simulink library "ddm"  (R2021b)
settings: Solver=VariableStepAuto  StartTime=0.0  StopTime=10.0  RelTol=1e-3
undefined symbols (not defined in the file or in its folder): ENUM_ADASACCSTA_ERROR, ENUM_ADASACCSTA_OFF, ENUM_ADASACCSTA_STANDBY, ENUM_ADASISASTA_OFF, ENUM_ALLOWMOV_ALLOWREADY, ENUM_APS, ENUM_BRKSTA_ERROR, ENUM_BRKSTA_OFF, ENUM_BRKSTA_ON, ENUM_CHGPREACTERRSTA_OBCPRE, ENUM_DCDCFAULTSTA_ANYFAULTLV1, ENUM_DCDCFAULTSTA_ANYFAULTLV2, ENUM_DRIVETRAIN_AWD, ENUM_DRIVETRAIN_FWD, ENUM_DRIVETRAIN_RWD, ENUM_DRSEATSTA_INVALID, ENUM_EDUDRTSTA_NORMAL, ENUM_EPBSTA_APPLIED, ENUM_EPBSTA_RELEASED, ENUM_HVBATTREADYPRE_READY, ENUM_MCUWARN_LV0, ENUM_MCUWARN_LV1, ENUM_MCUWARN_LV2, ENUM_MCUWARN_LV3, ENUM_MCUWARN_NOERROR, ENUM_OBCFAULTSTA_ANYFAULT, ENUM_PAS_R2F2, ENUM_PDFAULT_BATTPDFAIL, ENUM_PDFAULT_DCDCDISABLE, ENUM_PDFAULT_MCUDISABLE, ENUM_PDFAULT_MCUDISCHRG, ENUM_POWERSTA_OFF, ENUM_POWERSTA_ON, ENUM_POWERSTA_READY, ENUM_POWERSTA_STANDBY, ENUM_PRESSINDI_LOW, ENUM_PUFAULT_BATTUPFAIL, ENUM_PUFAULT_DCDCENABLEFAIL, ENUM_PUFAULT_PRECHRGCHKFAIL, ENUM_PUFAULT_SAFETYCHKFAIL, ENUM_PUSTATE_COMPLETED, ENUM_PWRSTASW_OFF, ENUM_PWRSTASW_OFFA, ENUM_PWRSTASW_OFFCHVCHRG, ENUM_PWRSTASW_OFFCLVCHRG, ENUM_PWRSTASW_ON, ENUM_PWRSTASW_ONHVCHRG, ENUM_PWRSTASW_READY, ENUM_PWRSTASW_STANDBY, ENUM_RANGESTA_12IN, ENUM_RANGESTA_12OUT, ENUM_SHIFTCOMMAND_D, ENUM_SHIFTCOMMAND_N, ENUM_SHIFTCOMMAND_P, ENUM_SHIFTCOMMAND_R, ENUM_ZONEMALFUNLV_1ST, ENUM_ZONEMALFUNLV_2ND, ENUM_ZONEMALFUNLV_3RD, ENUM_ZONEMALFUNLV_4TH, ENUM_ZONESPDCTRLMODE_ACC ... (+832)
libraries: hcu_lib x738, $bdroot x26, simulink x7
(part 8 of 25)

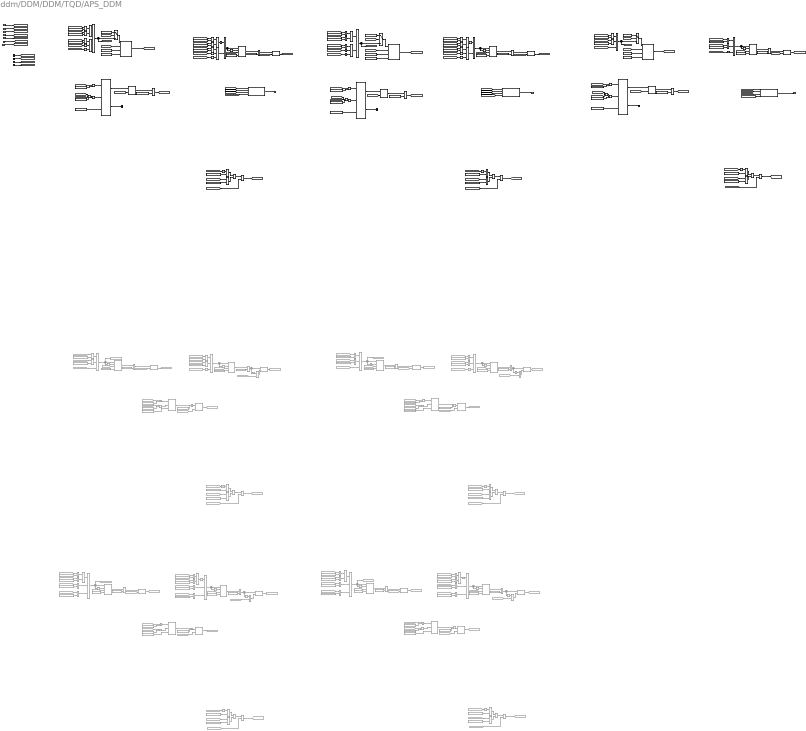
== system ddm/DDM/DDM/TQD/APS_DDM ==
  note: APS1 Signal Out of Range (APS1SigOoR)
  note: APS1_5V PWR Error (5vAPS1PwrErr)
  note: APS1 5V Out of Range (5vAPS1OoR)
  note: APS Correlation Error (APSCorrErr)
  note: APS2_5V PWR Error (5vAPS2PwrErr)
  note: APS2 Signal Out of Range (APS2SigOoR)
  note: APS2 5V Out of Range (5vAPS2OoR)
  VPMM_SysPwrSta_enum : Inport
  VINP_AccelPedal1Vol_V : Inport  Port=2
  VINP_AccelPedal2Vol_V : Inport  Port=3
  VDHP_EAPS12RangeSta_enum : Inport  Port=4
  VDHP_EAPCRBAD_flg : Inport  Port=5
  task_time_s : Inport  Port=6
  DTC_clear_request : Inport  Port=7
  Constant1 : Constant  Commented=on  Value=KDDM_5vAPS1PwrErrPassTO_ms
  Constant10 : Constant  Value=ENUM_POWERSTA_OFF
  Constant{62,65,84,92,100,103} (6 alike) : Constant  Value=ENUM_PWRSTASW_OFF
  Constant101 : Constant  Value=KDDM_APS2SigOoRHiLim_V
  Constant102 : Constant  Value=KDDM_APS2SigOoRLoLim_V
  Constant104 : Constant  Value=KDDM_APS2SigOoRHiLim_V
  Constant105 : Constant  Value=KDDM_APS2SigOoRLoLim_V
  Constant107 : Constant  Value=KDDM_APS2SigOoRPassTO_s
  Constant108 : Constant  Value=KDDM_APS2SigOoRPassTO_s
  Constant11 : Constant  Value=ENUM_POWERSTA_STANDBY
  Constant110 : Constant  Value=KDDM_APS2SigOoRCFSSW_flg
  Constant{16,20,22,72,75,79,82,111} (8 alike) : Constant  Commented=on  Value=KDDM_5vAPSErrBattSOC_pct
  Constant{9,21,32,42,44,54,112,114} (8 alike) : Constant  Commented=on  Value=ENUM_PWRSTASW_OFF
  Constant113 : Constant  Commented=on  Value=KDDM_5vAPS2PwrErrPassTO_ms
  Constant12 : Constant  Value=KDDM_APS1SigOoRDetSW_flg
  Constant13 : Constant  Value=KDDM_APS1SigOoRPassSW_flg
  Constant132 : Constant  Value=KDDM_APS1SigOoRDTC_cnt
  Constant14 : Constant  Value=KDDM_APS1SigOoRDTC_cnt
  Constant15 : Constant  Value=KDDM_APS2SigOoRDTC_cnt
  Constant17 : Constant  Commented=on  Value=KDDM_5vAPS1PwrErrDetTO_ms
  Constant18 : Constant  Commented=on  Value=KDDM_5vAPS1PwrErrDetTO_ms
  Constant19 : Constant  Commented=on  Value=KDDM_5vAPS2PwrErrPassTO_ms
  Constant{2,25,35,47} (4 alike) : Constant  Commented=on  Value=ENUM_POWERSTA_OFF
  Constant23 : Constant  Commented=on  Value=KDDM_5vAPS2PwrErrDetTO_ms
  Constant24 : Constant  Commented=on  Value=KDDM_5vAPS2PwrErrDetTO_ms
  Constant{3,26,36,48} (4 alike) : Constant  Commented=on  Value=ENUM_POWERSTA_STANDBY
  Constant27 : Constant  Commented=on  Value=KDDM_5vAPS2PwrErrDetSW_flg
  Constant28 : Constant  Commented=on  Value=KDDM_5vAPS2PwrErrPassSW_flg
  Constant29 : Constant  Commented=on  Value=KDDM_5vAPS2PwrErrDTC_cnt
  Constant30 : Constant  Commented=on  Value=KDDM_5vAPS2PwrErrDTC_cnt
  Constant{31,33..34,41} (4 alike) : Constant  Commented=on  Value=KDDM_5vAPS1OoRDetTO_ms
  Constant37 : Constant  Commented=on  Value=KDDM_5vAPS1OoRDetSW_flg
  Constant38 : Constant  Commented=on  Value=KDDM_5vAPS1OoRPassSW_flg
  Constant39 : Constant  Commented=on  Value=KDDM_5vAPS1OoRDTC_cnt
  Constant4 : Constant  Commented=on  Value=KDDM_5vAPS1PwrErrDetSW_flg
  Constant40 : Constant  Commented=on  Value=KDDM_5vAPS1OoRDTC_cnt
  Constant43 : Constant  Commented=on  Value=KDDM_5vAPS2OoRPassTO_ms
  Constant45 : Constant  Commented=on  Value=KDDM_5vAPS2OoRDetTO_ms
  Constant46 : Constant  Commented=on  Value=KDDM_5vAPS2OoRDetTO_ms
  Constant49 : Constant  Commented=on  Value=KDDM_5vAPS2OoRDetSW_flg
  Constant5 : Constant  Commented=on  Value=KDDM_5vAPS1PwrErrPassSW_flg
  Constant50 : Constant  Commented=on  Value=KDDM_5vAPS2OoRPassSW_flg
  Constant51 : Constant  Commented=on  Value=KDDM_5vAPS2OoRDTC_cnt
  Constant52 : Constant  Commented=on  Value=KDDM_5vAPS2OoRDTC_cnt
  Constant53 : Constant  Commented=on  Value=KDDM_5vAPS2OoRPassTO_ms
  Constant55 : Constant  Value=KDDM_APSCorrErrPassTO_s
  Constant56 : Constant  Value=ENUM_RANGESTA_12IN
  Constant57 : Constant  Value=KDDM_APSCorrErrDetTO_s
  Constant58 : Constant  Value=KDDM_APSCorrErrDTC_cnt
  Constant59 : Constant  Value=ENUM_POWERSTA_OFF
  Constant6 : Constant  Commented=on  Value=KDDM_5vAPS1PwrErrDTC_cnt
  Constant60 : Constant  Commented=on  Value=KDDM_5vAPS1OoRHiLim_V
  Constant61 : Constant  Commented=on  Value=KDDM_5vAPS1OoRLoLim_V
  Constant63 : Constant  Value=KDDM_APS1SigOoRHiLim_V
  Constant64 : Constant  Value=KDDM_APS1SigOoRLoLim_V
  Constant66 : Constant  Value=KDDM_APS1SigOoRHiLim_V
  Constant67 : Constant  Value=KDDM_APS1SigOoRLoLim_V
  Constant68 : Constant  Value=KDDM_APS2SigOoRDetTO_s
  Constant69 : Constant  Value=KDDM_APS1SigOoRPassTO_s
  Constant7 : Constant  Commented=on  Value=KDDM_5vAPS1PwrErrDTC_cnt
  Constant70 : Constant  Value=KDDM_APS1SigOoRPassTO_s
  Constant71 : Constant  Value=KDDM_APSCorrErrCFSSW_flg
  Constant73 : Constant  Commented=on  Value=KDDM_5vAPS1OoRHiLim_V
  Constant74 : Constant  Commented=on  Value=KDDM_5vAPS1OoRLoLim_V
  Constant76 : Constant  Value=ENUM_POWERSTA_STANDBY
  Constant77 : Constant  Commented=on  Value=KDDM_5vAPS2OoRHiLim_V
  Constant78 : Constant  Commented=on  Value=KDDM_5vAPS2OoRLoLim_V
  Constant8 : Constant  Commented=on  Value=KDDM_5vAPS1PwrErrPassTO_ms
  Constant80 : Constant  Commented=on  Value=KDDM_5vAPS2OoRHiLim_V
  Constant81 : Constant  Commented=on  Value=KDDM_5vAPS2OoRLoLim_V
  Constant83 : Constant  Value=ENUM_RANGESTA_12IN
  Constant85 : Constant  Value=FALSE
  Constant86 : Constant  Value=KDDM_APS1SigOoRDetTO_s
  Constant87 : Constant  Value=KDDM_APSCorrErrDetSW_flg
  Constant88 : Constant  Value=KDDM_APSCorrErrPassSW_flg
  Constant89 : Constant  Value=KDDM_APSCorrErrDTC_cnt
  Constant90 : Constant  Value=FALSE
  Constant91 : Constant  Value=KDDM_APSCorrErrPassTO_s
  Constant93 : Constant  Value=KDDM_APS1SigOoRCFSSW_flg
  Constant94 : Constant  Value=ENUM_POWERSTA_OFF
  Constant95 : Constant  Value=ENUM_POWERSTA_STANDBY
  Constant96 : Constant  Value=KDDM_APS2SigOoRDetSW_flg
  Constant97 : Constant  Value=KDDM_APS2SigOoRPassSW_flg
  Constant98 : Constant  Value=KDDM_APS2SigOoRDTC_cnt
  Constant99 : Constant  Value=FALSE
  Counter{1..4} (4 alike) : hcu_lib/Basic_Blocks/Counter  Commented=on
  DTC_Couter1 : hcu_lib/Basic_Blocks/DTC_Couter
  DTC_Couter2 : hcu_lib/Basic_Blocks/DTC_Couter
  DTC_Couter3 : hcu_lib/Basic_Blocks/DTC_Couter
  DTC_Info : hcu_lib/Basic_Blocks/DTC_Info
  DTC_Info1 : hcu_lib/Basic_Blocks/DTC_Info
  DTC_Info2 : hcu_lib/Basic_Blocks/DTC_Info
  Equal{1..2,11,13,18,30,34,39} (8 alike) : RelationalOperator  Commented=on  Operator=~=  OutDataTypeStr=boolean  RndMeth=Simplest
  Equal{6..7,10,12,14,16,38,40..41,47..49} (12 alike) : RelationalOperator  Commented=on  OutDataTypeStr=boolean  RndMeth=Simplest
  Equal{15,17,19,29,31,33,35,37,44,46,69..70} (12 alike) : RelationalOperator  Commented=on  Operator=>  OutDataTypeStr=boolean  RndMeth=Simplest
  Equal{20,32,36,45} (4 alike) : RelationalOperator  Commented=on  Operator=<  OutDataTypeStr=boolean  RndMeth=Simplest
  Equal{21,24,51,53,58,61} (6 alike) : RelationalOperator  Operator=~=  OutDataTypeStr=boolean  RndMeth=Simplest
  Equal{22,25,59,62} (4 alike) : RelationalOperator  Operator=>  OutDataTypeStr=boolean  RndMeth=Simplest
  Equal{23,26,60,63} (4 alike) : RelationalOperator  Operator=<  OutDataTypeStr=boolean  RndMeth=Simplest
  Equal28 : RelationalOperator  OutDataTypeStr=boolean  RndMeth=Simplest
  Equal{3..4,56..57,66..67,74..75} (8 alike) : RelationalOperator  Operator===  OutDataTypeStr=boolean  RndMeth=Simplest
  Equal{8..9,42..43,50,71..73} (8 alike) : RelationalOperator  Commented=on  Operator===  OutDataTypeStr=boolean  RndMeth=Simplest
  Equal55 : RelationalOperator  OutDataTypeStr=boolean  RndMeth=Simplest
  Equal65 : RelationalOperator  OutDataTypeStr=boolean  RndMeth=Simplest
  From : From  Commented=on  GotoTag=VDDM_5vAPS1PwrErrDet_flg
  From1 : From  Commented=on  GotoTag=VDDM_5vAPS1PwrErr_flg
  From{3,8..10,17,29,34,37,41,46,52,55,60,108,121,124} (16 alike) : From  Commented=on  GotoTag=VPMM_SysPwrSta_enum
  From104 : From  Commented=on  GotoTag=VDDM_5vAPS1OoRRst_flg
  From{42,47,105..106} (4 alike) : From  Commented=on  GotoTag=VINP_5vAPS1ADC_V
  From{4,25,30,36,51,54,107,120} (8 alike) : From  Commented=on  GotoTag=VINP_HVBattSOC_pct
  From{5..6,31..32,43..44,109..110} (8 alike) : From  Commented=on  GotoTag=task_time_s
  From11 : From  Commented=on  GotoTag=VDDM_5vAPS1PwrErrPass_flg
  From111 : From  Commented=on  GotoTag=VDDM_5vAPS2OoRPass_flg
  From12 : From  Commented=on  GotoTag=VDDM_5vAPS1PwrErrCFSRls_flg
  From{49..50,61,128} (4 alike) : From  Commented=on  GotoTag=VINP_5vAPS2ADC_V
  From13 : From  Commented=on  GotoTag=VDDM_5vAPS1PwrErrRst_flg
  From{14,27,40,59} (4 alike) : From  Commented=on  GotoTag=DTC_clear_request
  From15 : From  Commented=on  GotoTag=VDDM_5vAPS2PwrErrDet_flg
  From16 : From  Commented=on  GotoTag=VDDM_5vAPS2PwrErr_flg
  From18 : From  Commented=on  GotoTag=VDDM_5vAPS2PwrErrPass_flg
  From2 : From  Commented=on  GotoTag=VDDM_5vAPS1PwrErr_flg
  From23 : From  Commented=on  GotoTag=VDDM_5vAPS2PwrErrCFSRls_flg
  From26 : From  Commented=on  GotoTag=VDDM_5vAPS2PwrErrRst_flg
  From28 : From  Commented=on  GotoTag=VDDM_5vAPS2PwrErr_flg
  From33 : From  Commented=on  GotoTag=VDDM_5vAPS2PwrErrPass_flg
  From35 : From  Commented=on  GotoTag=VDDM_5vAPS1OoRDet_flg
  From38 : From  Commented=on  GotoTag=VDDM_5vAPS1OoRPass_flg
  From39 : From  Commented=on  GotoTag=VDDM_APS1SigErrCFSRls_flg
  From45 : From  Commented=on  GotoTag=VDDM_5vAPS1OoRPass_flg
  From48 : From  Commented=on  GotoTag=VDDM_5vAPS2OoRRst_flg
  From53 : From  Commented=on  GotoTag=VDDM_5vAPS2OoRDet_flg
  From57 : From  Commented=on  GotoTag=VDDM_5vAPS2OoRPass_flg
  From58 : From  Commented=on  GotoTag=VDDM_5vAPS2OoRCFSRls_flg
  From7 : From  Commented=on  GotoTag=VDDM_5vAPS1PwrErrPass_flg
  Goto : Goto  Commented=on  GotoTag=VDDM_5vAPS1PwrErrRst_flg
  Goto1 : Goto  Commented=on  GotoTag=VDDM_5vAPS1PwrErrDet_flg
  Goto10 : Goto  Commented=on  GotoTag=VDDM_5vAPS2PwrErrCFSRls_flg
  Goto11 : Goto  Commented=on  GotoTag=VDDM_5vAPS1OoRDet_flg
  Goto12 : Goto  Commented=on  GotoTag=VDDM_5vAPS1OoRPass_flg
  Goto13 : Goto  Commented=on  GotoTag=VDDM_APS1SigErrCFSRls_flg
  Goto14 : Goto  Commented=on  GotoTag=VDDM_5vAPS1OoRConfirm_flg
  Goto15 : Goto  Commented=on  GotoTag=VDDM_5vAPS2OoRPass_flg
  Goto16 : Goto  Commented=on  GotoTag=VDDM_5vAPS2OoRCFSRls_flg
  Goto17 : Goto  Commented=on  GotoTag=VDDM_5vAPS2OoRConfirm_flg
  Goto18 : Goto  Commented=on  GotoTag=VDDM_5vAPS2OoRRst_flg
  Goto2 : Goto  Commented=on  GotoTag=VDDM_5vAPS2OoRDet_flg
  Goto24 : Goto  Commented=on  GotoTag=VDDM_5vAPS1OoRRst_flg
  Goto27 : Goto  Commented=on  GotoTag=VDDM_5vAPS1PwrErrPass_flg
  Goto3 : Goto  Commented=on  GotoTag=VDDM_5vAPS1PwrErrCFSRls_flg
  Goto33 : Goto  Commented=on  GotoTag=VDDM_5vAPS2PwrErrConfirm_flg
  Goto4 : Goto  Commented=on  GotoTag=VDDM_5vAPS1PwrErrConfirm_flg
  Goto5 : Goto  Commented=on  GotoTag=VDDM_5vAPS2PwrErrRst_flg
  Goto6 : Goto  Commented=on  GotoTag=VDDM_5vAPS2PwrErrDet_flg
  Goto7 : Goto  Commented=on  GotoTag=VDDM_5vAPS2PwrErrPass_flg
  Ground{3..6} (4 alike) : Ground
  Logical Operator{,1..2,10,18..19,25..26,46..47,49..50} (12 alike) : Logic  Commented=on  Operator=OR  AllPortsSameDT=off  OutDataTypeStr=boolean
  Logical Operator{30,38,70,86,100,107} (6 alike) : Logic  Inputs=3  AllPortsSameDT=off  OutDataTypeStr=boolean
  Logical Operator{4..6,31..32,34,39,82,84..85,101..102,108..109,115..116} (16 alike) : Logic  AllPortsSameDT=off  OutDataTypeStr=boolean
  Logical Operator{12,33,35,41,43,60,80,97,103,110} (10 alike) : Logic  Operator=OR  AllPortsSameDT=off  OutDataTypeStr=boolean
  Logical Operator{28..29,36..37,42,71,73,83,98..99,105..106,111..112} (14 alike) : Logic  Operator=NOT  AllPortsSameDT=off  OutDataTypeStr=boolean
  Logical Operator{8..9,11,14,17,21,27,45,51,53..54,58,63..65,69} (16 alike) : Logic  Commented=on  Operator=NOT  AllPortsSameDT=off  OutDataTypeStr=boolean
  Logical Operator{13,15..16,20,22..24,48,55..56,66..67} (12 alike) : Logic  Commented=on  AllPortsSameDT=off  OutDataTypeStr=boolean
  Logical Operator{3,7,44,52,57,61..62,68} (8 alike) : Logic  Commented=on  Inputs=3  AllPortsSameDT=off  OutDataTypeStr=boolean
  SR_Latch{,6,12,15,18,20} (6 alike) : hcu_lib/Basic_Blocks/SR_Latch
  SR_Latch{1..5,7..11,16..17} (12 alike) : hcu_lib/Basic_Blocks/SR_Latch  Commented=on
  Switch1 : Switch  Criteria=u2 ~= 0
  Switch2 : Switch  Criteria=u2 ~= 0
  Switch6 : Switch  Criteria=u2 ~= 0
  Terminator : Terminator
  Terminator1 : Terminator
  Terminator2 : Terminator
  Test Detection Criteria1 : hcu_lib/Basic_Blocks/Test Detection Criteria
  Test Detection Criteria3 : hcu_lib/Basic_Blocks/Test Detection Criteria
  Test Detection Criteria4 : hcu_lib/Basic_Blocks/Test Detection Criteria
  Timer1 : hcu_lib/Basic_Blocks/Timer
  Timer13 : hcu_lib/Basic_Blocks/Timer
  Timer15 : hcu_lib/Basic_Blocks/Timer
  Timer{2..9} (8 alike) : hcu_lib/Basic_Blocks/Timer  Commented=on
  Unit Delay : UnitDelay  SampleTime=-1  HasFrameUpgradeWarning=on
  Unit Delay{1..4} (4 alike) : UnitDelay  Commented=on  SampleTime=-1  HasFrameUpgradeWarning=on
  Unit Delay5 : UnitDelay  SampleTime=-1  HasFrameUpgradeWarning=on
  Unit Delay7 : UnitDelay  SampleTime=-1  HasFrameUpgradeWarning=on
  VDDM_APS1SigOoRDTC_raw32 : Outport
  VDDM_APS2SigOoRDTC_raw32 : Outport  Port=2
  VDDM_APSCorrErrDTC_raw32 : Outport  Port=3
  wires:
  [VDDM_APSCorrErrPass_flg] -> DTC_Info2/2
  [VDDM_APSCorrErrDet_flg] -> DTC_Info2/1
  [VDDM_APS2SigOoRPass_flg] -> DTC_Info1/2
  [VDDM_APS2SigOoRDet_flg] -> DTC_Info1/1
  [VDDM_APS1SigOoRDet_flg] -> DTC_Info/1
  DTC_clear_request/1 -> [DTC_clear_request]
  Ground5/1 -> [VDDM_5vAPS2OoRCFS_flg]
  Ground6/1 -> [VDDM_5vAPS2PwrErrCFS_flg]
  task_time_s/1 -> [task_time_s]
  Ground4/1 -> [VDDM_5vAPS1PwrErrCFS_flg]
  Ground3/1 -> [VDDM_5vAPS1OoRCFS_flg]
  [VPMM_SysPwrSta_enum] -> Unit Delay/1
  Unit Delay/1 -> Equal3/1
  Constant10/1 -> Equal3/2
  Constant11/1 -> Equal4/2
  [VPMM_SysPwrSta_enum] -> Equal4/1
  Equal3/1 -> Logical Operator4/1
  Equal4/1 -> Logical Operator4/2
  [VDDM_APS1SigOoRDet_flg] -> Logical Operator5/1
  Constant12/1 -> Logical Operator5/2
  Constant13/1 -> Logical Operator6/2
  [DTC_clear_request] -> Logical Operator12/2
  Logical Operator4/1 -> Logical Operator12/1
  Logical Operator12/1 -> [VDDM_APS1SigOoRCFSRls_flg]
  Logical Operator30/1 -> Logical Operator31/2
  Logical Operator29/1 -> Logical Operator30/3
  Logical Operator28/1 -> Logical Operator30/2
  Equal21/1 -> Logical Operator30/1
  [VDDM_5vAPS1PwrErrCFS_flg] -> Logical Operator29/1
  [VDDM_5vAPS1OoRCFS_flg] -> Logical Operator28/1
  Constant62/1 -> Equal21/2
  [VPMM_SysPwrSta_enum] -> Equal21/1
  Equal23/1 -> Logical Operator33/2
  Equal22/1 -> Logical Operator33/1
  Constant64/1 -> Equal23/2
  Constant63/1 -> Equal22/2
  [VINP_AccelPedal1Vol_V] -> Equal23/1
  [VINP_AccelPedal1Vol_V] -> Equal22/1
  Logical Operator33/1 -> Logical Operator31/1
  Logical Operator41/1 -> Logical Operator42/1
  [VINP_AccelPedal1Vol_V] -> Equal25/1
  [VINP_AccelPedal1Vol_V] -> Equal26/1
  Constant66/1 -> Equal25/2
  Constant67/1 -> Equal26/2
  Equal25/1 -> Logical Operator41/1
  Equal26/1 -> Logical Operator41/2
  [VPMM_SysPwrSta_enum] -> Equal24/1
  Constant65/1 -> Equal24/2
  [VDDM_5vAPS1OoRCFS_flg] -> Logical Operator36/1
  [VDDM_5vAPS1PwrErrCFS_flg] -> Logical Operator37/1
  Equal24/1 -> Logical Operator38/1
  Logical Operator36/1 -> Logical Operator38/2
  Logical Operator37/1 -> Logical Operator38/3
  Logical Operator38/1 -> Logical Operator39/2
  Logical Operator42/1 -> Logical Operator39/1
  Logical Operator73/1 -> Timer1/2
  Constant69/1 -> Equal28/2
  Timer1/1 -> Equal28/1
  Constant70/1 -> Timer1/4
  [task_time_s] -> Timer1/3
  Constant18/1 -> Timer4/4
  From7/1 -> SR_Latch2/2
  Constant7/1 -> Equal10/2
  Constant2/1 -> Equal8/2
  Timer5/1 -> Equal7/1
  Constant8/1 -> Equal7/2
  From/1 -> Logical Operator15/1
  Logical Operator7/1 -> Goto/1, Logical Operator8/1, Timer4/1
  From3/1 -> Equal1/1
  From6/1 -> Timer5/3
  Constant6/1 -> Counter1/3
  SR_Latch2/1 -> Goto1/1
  Equal10/1 -> SR_Latch1/1
  Logical Operator14/1 -> Timer5/2
  From10/1 -> Equal9/1
  Constant3/1 -> Equal9/2
  Equal1/1 -> Logical Operator7/1
  From12/1 -> SR_Latch1/2
  Constant1/1 -> Timer5/4
  Constant9/1 -> Equal1/2
  Constant5/1 -> Logical Operator16/2
  Constant17/1 -> Equal6/2
  Logical Operator15/1 -> Counter1/1
  Counter1/1 -> Equal10/1
  Equal8/1 -> Logical Operator13/1
  Timer4/1 -> Equal6/1
  Logical Operator8/1 -> Timer4/2
  From11/1 -> Logical Operator16/1
  From8/1 -> Unit Delay1/1
  Logical Operator16/1 -> Counter1/2
  From14/1 -> Logical Operator1/2
  Equal6/1 -> SR_Latch2/1
  From5/1 -> Timer4/3
  Logical Operator1/1 -> Goto3/1
  Equal9/1 -> Logical Operator13/2
  Logical Operator13/1 -> Logical Operator1/1
  SR_Latch1/1 -> Goto4/1
  Constant4/1 -> Logical Operator15/2
  Unit Delay1/1 -> Equal8/1
  Constant37/1 -> Logical Operator66/2
  Counter3/1 -> Equal38/1
  Constant34/1 -> Timer8/4
  From38/1 -> Logical Operator67/1
  Logical Operator69/1 -> Timer8/2
  From39/1 -> SR_Latch5/2
  Equal40/1 -> SR_Latch9/1
  Constant41/1 -> Equal41/2
  Logical Operator68/1 -> Goto24/1, Logical Operator69/1, Timer8/1
  Constant42/1 -> Equal18/2
  From45/1 -> SR_Latch9/2
  From35/1 -> Logical Operator66/1
  From43/1 -> Timer8/3
  SR_Latch9/1 -> Goto11/1
  Constant40/1 -> Equal38/2
  From41/1 -> Equal18/1
  Equal38/1 -> SR_Latch5/1
  Timer8/1 -> Equal40/1
  From44/1 -> Timer9/3
  Equal18/1 -> Logical Operator68/2
  Logical Operator44/1 -> Timer9/1, Logical Operator65/1
  Logical Operator65/1 -> Timer9/2
  Logical Operator66/1 -> Counter3/1
  Logical Operator67/1 -> Counter3/2
  Timer9/1 -> Equal41/1
  Constant33/1 -> Equal40/2
  Constant31/1 -> Timer9/4
  Constant38/1 -> Logical Operator67/2
  Constant39/1 -> Counter3/3
  SR_Latch5/1 -> Goto14/1
  Constant35/1 -> Equal42/2
  From40/1 -> Logical Operator18/2
  Equal42/1 -> Logical Operator22/1
  Constant36/1 -> Equal43/2
  Equal43/1 -> Logical Operator22/2
  From46/1 -> Unit Delay3/1
  Logical Operator18/1 -> Goto13/1
  From37/1 -> Equal43/1
  Unit Delay3/1 -> Equal42/1
  Logical Operator22/1 -> Logical Operator18/1
  [VPMM_SysPwrSta_enum] -> Equal57/1
  [VPMM_SysPwrSta_enum] -> Unit Delay5/1
  Equal56/1 -> Logical Operator82/1
  Equal57/1 -> Logical Operator82/2
  [DTC_clear_request] -> Logical Operator80/2
  Constant57/1 -> Test Detection Criteria1/4
  [task_time_s] -> Timer13/3
  Constant59/1 -> Equal56/2
  [VDDM_APSCorrErrDet_flg] -> Logical Operator84/1
  Constant88/1 -> Logical Operator85/2
  Timer13/1 -> Equal55/1
  Logical Operator85/1 -> DTC_Couter3/2
  Logical Operator84/1 -> DTC_Couter3/1
  Logical Operator83/1 -> Timer13/2
  Test Detection Criteria1/1 -> [VDDM_APSCorrErrDet_flg]  "VDDM_APSCorrErrDet_flg"
  Unit Delay5/1 -> Equal56/1
  Constant91/1 -> Equal55/2
  [task_time_s] -> Test Detection Criteria1/2
  Logical Operator82/1 -> Logical Operator80/1
  [VDDM_APSCorrCFSRls_flg] -> SR_Latch12/2
  Logical Operator80/1 -> [VDDM_APSCorrCFSRls_flg]
  Constant87/1 -> Logical Operator84/2
  Constant55/1 -> Timer13/4
  Constant76/1 -> Equal57/2
  Equal51/1 -> Logical Operator86/1
  Constant92/1 -> Equal51/2
  [VPMM_SysPwrSta_enum] -> Equal51/1
  [VDHP_EAPCRBAD_flg] -> Logical Operator86/3
  SR_Latch/1 -> Logical Operator32/1
  Logical Operator32/1 -> [VDDM_APS1SigOoRCFS_flg]
  Constant93/1 -> Logical Operator32/2
  From120/1 -> Equal69/1
  Equal69/1 -> Logical Operator7/2
  Constant111/1 -> Equal69/2
  From1/1 -> Logical Operator7/3
  Constant16/1 -> Equal70/2
  From4/1 -> Equal70/1
  Equal70/1 -> Logical Operator3/2
  Equal2/1 -> Logical Operator3/1
  Logical Operator3/1 -> Logical Operator14/1, Timer5/1
  Constant112/1 -> Equal2/2
  From9/1 -> Equal2/1
  From2/1 -> Logical Operator9/1
  Logical Operator9/1 -> Logical Operator3/3
  SR_Latch16/1 -> Goto27/1
  Equal7/1 -> Logical Operator11/1, SR_Latch16/1
  From13/1 -> Logical Operator/2
  Logical Operator/1 -> SR_Latch16/2
  Logical Operator11/1 -> Logical Operator/1
  Equal72/1 -> Logical Operator20/2
  Equal11/1 -> Logical Operator62/1
  Equal71/1 -> Logical Operator20/1
  Logical Operator63/1 -> Timer6/2
  Logical Operator24/1 -> Counter2/2
  Constant19/1 -> Timer7/4
  Constant25/1 -> Equal71/2
  Constant23/1 -> Equal14/2
  From34/1 -> Unit Delay2/1
  Logical Operator62/1 -> Goto5/1, Logical Operator63/1, Timer6/1
  Counter2/1 -> Equal12/1
  From25/1 -> Equal15/1
  Unit Delay2/1 -> Equal71/1
  Constant24/1 -> Timer6/4
  Logical Operator17/1 -> Logical Operator2/1
  SR_Latch17/1 -> Goto6/1
  Constant28/1 -> Logical Operator24/2
  From26/1 -> Logical Operator2/2
  Logical Operator20/1 -> Logical Operator10/1
  From15/1 -> Logical Operator23/1
  SR_Latch4/1 -> Goto7/1
  Logical Operator64/1 -> Logical Operator61/3
  Timer6/1 -> Equal14/1
  Constant22/1 -> Equal17/2
  Logical Operator21/1 -> Timer7/2
  From16/1 -> Logical Operator62/3
  Equal17/1 -> Logical Operator61/2
  Constant26/1 -> Equal72/2
  From33/1 -> SR_Latch17/2
  Equal13/1 -> Logical Operator61/1
  From30/1 -> Equal17/1
  Constant29/1 -> Counter2/3
  Constant27/1 -> Logical Operator23/2
  From121/1 -> Equal13/1
  From17/1 -> Equal72/1
  Equal14/1 -> SR_Latch17/1
  From27/1 -> Logical Operator10/2
  Constant21/1 -> Equal13/2
  Logical Operator61/1 -> Logical Operator21/1, Timer7/1
  From18/1 -> Logical Operator24/1
  From28/1 -> Logical Operator64/1
  Constant20/1 -> Equal15/2
  From29/1 -> Equal11/1
  From32/1 -> Timer7/3
  Logical Operator2/1 -> SR_Latch4/2
  Timer7/1 -> Equal16/1
  Equal16/1 -> Logical Operator17/1, SR_Latch4/1
  From31/1 -> Timer6/3
  Equal12/1 -> SR_Latch3/1
  Logical Operator23/1 -> Counter2/1
  Constant114/1 -> Equal11/2
  Constant30/1 -> Equal12/2
  Constant113/1 -> Equal16/2
  Logical Operator10/1 -> Goto10/1
  SR_Latch3/1 -> Goto33/1
  Equal15/1 -> Logical Operator62/2
  From23/1 -> SR_Latch3/2
  SR_Latch18/1 -> [VDDM_APS1SigOoRPass_flg]
  [DTC_clear_request] -> Logical Operator97/2
  Constant95/1 -> Equal67/2
  Logical Operator108/1 -> Logical Operator112/1, Timer15/1
  Logical Operator100/1 -> Logical Operator101/2
  Equal67/1 -> Logical Operator109/2
  Logical Operator107/1 -> Logical Operator108/2
  Equal61/1 -> Logical Operator107/1
  Logical Operator103/1 -> Logical Operator101/1
  Equal58/1 -> Logical Operator100/1
  Constant94/1 -> Equal66/2
  Test Detection Criteria4/1 -> [VDDM_APS2SigOoRDet_flg]  "VDDM_APS2SigOoRDet_flg"
  Constant101/1 -> Equal59/2
  Logical Operator109/1 -> Logical Operator97/1
  Constant104/1 -> Equal62/2
  Logical Operator110/1 -> Logical Operator111/1
  Logical Operator98/1 -> Logical Operator100/2
  Logical Operator99/1 -> Logical Operator100/3
  Equal59/1 -> Logical Operator103/1
  Constant96/1 -> Logical Operator115/2
  Constant100/1 -> Equal58/2
  Constant97/1 -> Logical Operator116/2
  Constant107/1 -> Equal65/2
  [VPMM_SysPwrSta_enum] -> Unit Delay7/1
  Constant110/1 -> Logical Operator102/2
  Logical Operator102/1 -> [VDDM_APS2SigOoRCFS_flg]
  [VPMM_SysPwrSta_enum] -> Equal67/1
  Equal62/1 -> Logical Operator110/1
  Logical Operator111/1 -> Logical Operator108/1
  [VDDM_5vAPS2PwrErrCFS_flg] -> Logical Operator99/1
  Constant108/1 -> Timer15/4
  Constant103/1 -> Equal61/2
  Logical Operator112/1 -> Timer15/2
  Timer15/1 -> Equal65/1
  Equal63/1 -> Logical Operator110/2
  [VINP_AccelPedal2Vol_V] -> Equal63/1
  Equal60/1 -> Logical Operator103/2
  [VPMM_SysPwrSta_enum] -> Equal61/1
  [VPMM_SysPwrSta_enum] -> Equal58/1
  Logical Operator106/1 -> Logical Operator107/3
  Constant102/1 -> Equal60/2
  [VINP_AccelPedal2Vol_V] -> Equal62/1
  [VINP_AccelPedal2Vol_V] -> Equal59/1
  Constant105/1 -> Equal63/2
  Logical Operator105/1 -> Logical Operator107/2
  [VDDM_5vAPS2PwrErrCFS_flg] -> Logical Operator106/1
  [VDDM_5vAPS2OoRCFS_flg] -> Logical Operator105/1
  [VDDM_APS2SigOoRDet_flg] -> Logical Operator115/1
  Equal65/1 -> SR_Latch15/1
  Unit Delay7/1 -> Equal66/1
  Equal66/1 -> Logical Operator109/1
  SR_Latch15/1 -> [VDDM_APS2SigOoRPass_flg]
  [task_time_s] -> Timer15/3
  [VINP_AccelPedal2Vol_V] -> Equal60/1
  Logical Operator97/1 -> [VDDM_APS2SigOoRCFSRls_flg]
  [VDDM_5vAPS2OoRCFS_flg] -> Logical Operator98/1
  SR_Latch7/1 -> Goto12/1
  Constant61/1 -> Equal20/2
  Constant60/1 -> Equal19/2
  From106/1 -> Equal20/1
  Logical Operator25/1 -> Logical Operator68/1
  From105/1 -> Equal19/1
  Equal20/1 -> Logical Operator25/2
  Equal19/1 -> Logical Operator25/1
  Constant72/1 -> Equal29/2
  From36/1 -> Equal29/1
  Equal29/1 -> Logical Operator68/3
  Equal41/1 -> Logical Operator27/1, SR_Latch7/1
  From104/1 -> Logical Operator26/2
  Logical Operator27/1 -> Logical Operator26/1
  Logical Operator26/1 -> SR_Latch7/2
  Equal33/1 -> Logical Operator44/3
  Constant75/1 -> Equal33/2
  Equal32/1 -> Logical Operator19/2
  From42/1 -> Equal31/1
  Equal31/1 -> Logical Operator19/1
  From47/1 -> Equal32/1
  Constant74/1 -> Equal32/2
  Constant32/1 -> Equal30/2
  Equal30/1 -> Logical Operator44/2
  From107/1 -> Equal33/1
  From108/1 -> Equal30/1
  Constant73/1 -> Equal31/2
  Logical Operator45/1 -> Logical Operator44/1
  Logical Operator19/1 -> Logical Operator45/1
  Constant80/1 -> Equal44/2
  From54/1 -> Equal37/1
  Constant46/1 -> Timer2/4
  Logical Operator56/1 -> Counter4/2
  Constant49/1 -> Logical Operator55/2
  Logical Operator53/1 -> Logical Operator52/1
  Timer2/1 -> Equal48/1
  SR_Latch10/1 -> Goto15/1
  Equal48/1 -> SR_Latch11/1
  Logical Operator49/1 -> Logical Operator57/1
  Constant79/1 -> Equal37/2
  Constant48/1 -> Equal73/2
  From50/1 -> Equal36/1
  Equal35/1 -> Logical Operator49/1
  Equal37/1 -> Logical Operator57/3
  Equal49/1 -> Logical Operator51/1, SR_Latch10/1
  Constant52/1 -> Equal47/2
  Logical Operator52/1 -> Timer3/1, Logical Operator54/1
  From124/1 -> Unit Delay4/1
  From48/1 -> Logical Operator50/2
  Equal73/1 -> Logical Operator48/2
  From58/1 -> SR_Latch8/2
  Equal44/1 -> Logical Operator47/1
  Logical Operator50/1 -> SR_Latch10/2
  Constant82/1 -> Equal46/2
  Constant81/1 -> Equal45/2
  Constant78/1 -> Equal36/2
  Equal36/1 -> Logical Operator49/2
  From59/1 -> Logical Operator46/2
  Constant53/1 -> Equal49/2
  From51/1 -> Equal46/1
  Equal50/1 -> Logical Operator48/1
  Logical Operator46/1 -> Goto16/1
  Logical Operator51/1 -> Logical Operator50/1
  Logical Operator48/1 -> Logical Operator46/1
  From128/1 -> Equal45/1
  From53/1 -> Logical Operator55/1
  From55/1 -> Equal73/1
  Unit Delay4/1 -> Equal50/1
  From109/1 -> Timer2/3
  Equal39/1 -> Logical Operator52/2
  Logical Operator47/1 -> Logical Operator53/1
  Timer3/1 -> Equal49/1
  From57/1 -> Logical Operator56/1
  Equal45/1 -> Logical Operator47/2
  Constant54/1 -> Equal34/2
  From111/1 -> SR_Latch11/2
  Counter4/1 -> Equal47/1
  Equal46/1 -> Logical Operator52/3
  Equal34/1 -> Logical Operator57/2
  Logical Operator58/1 -> Timer2/2
  From60/1 -> Equal34/1
  Logical Operator54/1 -> Timer3/2
  Constant51/1 -> Counter4/3
  Constant47/1 -> Equal50/2
  Constant43/1 -> Timer3/4
  From49/1 -> Equal35/1
  Constant45/1 -> Equal48/2
  Logical Operator57/1 -> Goto18/1, Logical Operator58/1, Timer2/1
  SR_Latch11/1 -> Goto2/1
  Constant44/1 -> Equal39/2
  Constant50/1 -> Logical Operator56/2
  From52/1 -> Equal39/1
  Equal47/1 -> SR_Latch8/1
  Logical Operator55/1 -> Counter4/1
  From110/1 -> Timer3/3
  From61/1 -> Equal44/1
  SR_Latch8/1 -> Goto17/1
  Constant77/1 -> Equal35/2
  SR_Latch20/1 -> [VDDM_APSCorrErrPass_flg]
  Equal55/1 -> SR_Latch20/1
  [VDHP_EAPS12RangeSta_enum] -> Equal74/1
  Equal74/1 -> Logical Operator86/2
  Constant83/1 -> Equal74/2
  Equal75/1 -> Logical Operator70/2
  Equal53/1 -> Logical Operator70/1
  [VDHP_EAPS12RangeSta_enum] -> Equal75/1
  Logical Operator70/1 -> Logical Operator83/1, Timer13/1
  Constant56/1 -> Equal75/2
  [VPMM_SysPwrSta_enum] -> Equal53/1
  Constant84/1 -> Equal53/2
  [VDHP_EAPCRBAD_flg] -> Logical Operator71/1
  Logical Operator71/1 -> Logical Operator70/3
  [task_time_s] -> Test Detection Criteria3/2
  Constant86/1 -> Test Detection Criteria3/4
  Constant132/1 -> Test Detection Criteria3/3
  Test Detection Criteria3/1 -> [VDDM_APS1SigOoRDet_flg]  "VDDM_APS1SigOoRDet_flg"
  [VDDM_APS1SigOoRCFS_flg] -> DTC_Info/3
  [VDDM_APS1SigOoRPass_flg] -> DTC_Info/2
  DTC_Info/1 -> VDDM_APS1SigOoRDTC_raw32/1  "VDDM_APS1SigOoRDTC_raw32"
  Logical Operator5/1 -> DTC_Couter1/1
  Logical Operator6/1 -> DTC_Couter1/2
  Constant14/1 -> DTC_Couter1/3
  DTC_Couter1/1 -> SR_Latch/1
  [VDDM_APS1SigOoRCFSRls_flg] -> SR_Latch/2
  Logical Operator39/1 -> Timer1/1, Logical Operator73/1
  Equal28/1 -> SR_Latch18/1
  DTC_Couter1/2 -> Terminator/1  "VDDM_APS1SigOoRDTC_cnt"
  [task_time_s] -> Test Detection Criteria4/2
  Constant15/1 -> Test Detection Criteria4/3
  Constant68/1 -> Test Detection Criteria4/4
  Logical Operator115/1 -> DTC_Couter2/1
  Logical Operator116/1 -> DTC_Couter2/2
  Constant98/1 -> DTC_Couter2/3
  DTC_Couter2/2 -> Terminator1/1  "VDDM_APS2SigOoRDTC_cnt"
  DTC_Couter2/1 -> SR_Latch6/1
  [VDDM_APS2SigOoRCFSRls_flg] -> SR_Latch6/2
  SR_Latch6/1 -> Logical Operator102/1
  [VDDM_APS2SigOoRCFS_flg] -> DTC_Info1/3
  DTC_Info1/1 -> VDDM_APS2SigOoRDTC_raw32/1  "VDDM_APS2SigOoRDTC_raw32"
  VPMM_SysPwrSta_enum/1 -> [VPMM_SysPwrSta_enum]
  VINP_AccelPedal1Vol_V/1 -> [VINP_AccelPedal1Vol_V]
  VINP_AccelPedal2Vol_V/1 -> [VINP_AccelPedal2Vol_V]
  Constant58/1 -> Test Detection Criteria1/3
  Constant89/1 -> DTC_Couter3/3
  DTC_Couter3/1 -> SR_Latch12/1
  DTC_Couter3/2 -> Terminator2/1  "VDDM_APSCorrErrDTC_cnt"
  [VDDM_APSCorrErrCFS_flg] -> DTC_Info2/3
  DTC_Info2/1 -> VDDM_APSCorrErrDTC_raw32/1  "VDDM_APSCorrErrDTC_raw32"
  VDHP_EAPS12RangeSta_enum/1 -> [VDHP_EAPS12RangeSta_enum]
  VDHP_EAPCRBAD_flg/1 -> [VDHP_EAPCRBAD_flg]
  Constant71/1 -> Logical Operator34/2
  SR_Latch12/1 -> Logical Operator34/1
  Logical Operator34/1 -> [VDDM_APSCorrErrCFS_flg]
  [DTC_clear_request] -> DTC_Info/4
  [DTC_clear_request] -> DTC_Info1/4
  [DTC_clear_request] -> DTC_Info2/4
  [DTC_clear_request] -> Switch6/2
  Switch6/1 -> Test Detection Criteria3/1
  Logical Operator31/1 -> [VDDM_APS1SigOoRRst_flg], Switch6/3
  Constant85/1 -> Switch6/1
  [DTC_clear_request] -> Switch1/2
  Switch1/1 -> Test Detection Criteria4/1
  Logical Operator101/1 -> [VDDM_APS2SigOoRRst_flg], Switch1/3
  Constant90/1 -> Switch1/1
  [DTC_clear_request] -> Switch2/2
  Switch2/1 -> Test Detection Criteria1/1
  Logical Operator86/1 -> [VDDM_APSCorrErrRst_flg], Switch2/3
  Constant99/1 -> Switch2/1
  [VDDM_APS1SigOoRPass_flg] -> Logical Operator35/2
  [VDDM_APS1SigOoRCFSRls_flg] -> Logical Operator35/1
  Logical Operator35/1 -> Logical Operator6/1
  [VDDM_APS2SigOoRCFSRls_flg] -> Logical Operator43/1
  [VDDM_APS2SigOoRPass_flg] -> Logical Operator43/2
  Logical Operator43/1 -> Logical Operator116/1
  [VDDM_APSCorrCFSRls_flg] -> Logical Operator60/1
  [VDDM_APSCorrErrPass_flg] -> Logical Operator60/2
  Logical Operator60/1 -> Logical Operator85/1
  [VDDM_APS1SigOoRRst_flg] -> SR_Latch18/2
  [VDDM_APS2SigOoRRst_flg] -> SR_Latch15/2
  [VDDM_APSCorrErrRst_flg] -> SR_Latch20/2

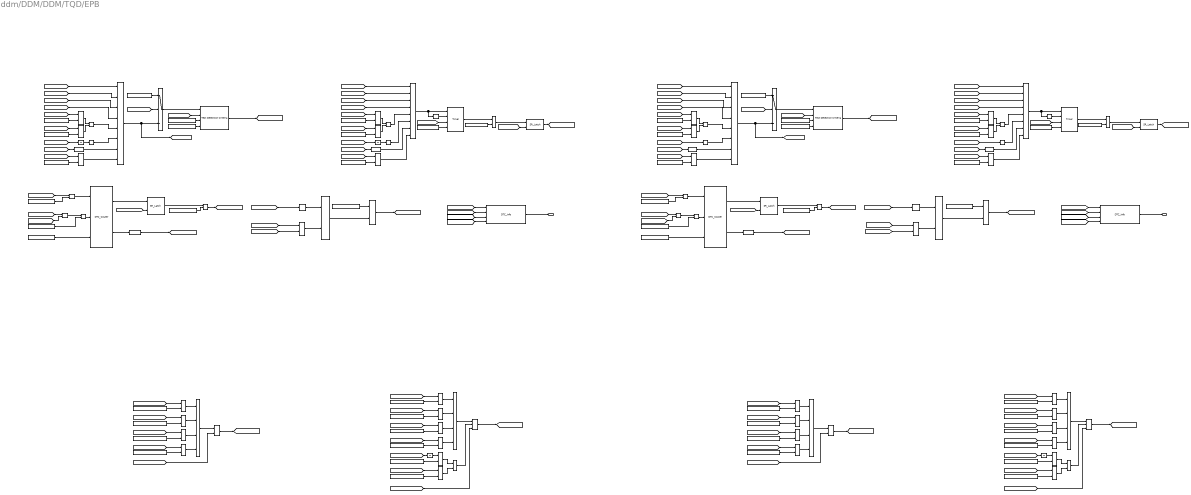
== system ddm/DDM/DDM/TQD/EPB ==
  note: EPB Apply Response Timeout (EPBLockTO)
  note: EPB Release Response Timeout (EPBUnlockTO)
  Constant{,3,23,39} (4 alike) : Constant  Value=ENUM_PWRSTASW_ON
  Constant1 : Constant  Value=KDDM_EPBLockTOCFSSW_flg
  Constant{8,10,25,49} (4 alike) : Constant  Value=ENUM_PWRSTASW_READY
  Constant11 : Constant  Value=ENUM_EPBSTA_APPLIED
  Constant12 : Constant  Value=ENUM_POWERSTA_OFF
  Constant13 : Constant  Value=ENUM_POWERSTA_STANDBY
  Constant{14,29,41,45} (4 alike) : Constant  Value=ENUM_SHIFTCOMMAND_P
  Constant15 : Constant  Value=KDDM_EPBLockTODTC_cnt
  Constant16 : Constant  Value=KDDM_EPBLockTODFSSW_flg
  Constant{17,32,42,46} (4 alike) : Constant  Value=ENUM_SHIFTCOMMAND_N
  Constant{4,18,33,40} (4 alike) : Constant  Value=ENUM_SHIFTCOMMAND_D
  Constant{5,19,34,43} (4 alike) : Constant  Value=ENUM_SHIFTCOMMAND_R
  Constant2 : Constant  Value=FALSE
  Constant20 : Constant  Value=KDDM_EPBLockTODTC_cnt
  Constant21 : Constant  Value=KDDM_EPBLockTOPassTO_s
  Constant22 : Constant  Value=KDDM_EPBLockTODetTO_s
  Constant24 : Constant  Value=KDDM_EPBUnlockTOCFSSW_flg
  Constant26 : Constant  Value=ENUM_EPBSTA_RELEASED
  Constant27 : Constant  Value=ENUM_POWERSTA_OFF
  Constant28 : Constant  Value=ENUM_POWERSTA_STANDBY
  Constant30 : Constant  Value=KDDM_EPBUnlockTODTC_cnt
  Constant31 : Constant  Value=KDDM_EPBUnlockTODFSSW_flg
  Constant35 : Constant  Value=FALSE
  Constant36 : Constant  Value=KDDM_EPBUnlockTODTC_cnt
  Constant37 : Constant  Value=KDDM_EPBUnlockTOPassTO_s
  Constant38 : Constant  Value=KDDM_EPBUnlockTODetTO_s
  Constant44 : Constant  Value=KDDM_EPBUnlockTODetSW_flg
  Constant47 : Constant  Value=KDDM_EPBUnlockTOPassSW_flg
  Constant48 : Constant  Value=KDDM_EPBUnlockTOPassTO_s
  Constant50 : Constant  Value=ENUM_EPBSTA_RELEASED
  Constant6 : Constant  Value=KDDM_EPBLockTODetSW_flg
  Constant7 : Constant  Value=KDDM_EPBLockTOPassSW_flg
  Constant70 : Constant  Value=KDDM_EPBLockTOPassTO_s
  Constant9 : Constant  Value=ENUM_EPBSTA_APPLIED
  DTC_Couter1 : hcu_lib/Basic_Blocks/DTC_Couter
  DTC_Couter2 : hcu_lib/Basic_Blocks/DTC_Couter
  DTC_Info : hcu_lib/Basic_Blocks/DTC_Info
  DTC_Info1 : hcu_lib/Basic_Blocks/DTC_Info
  Data Type Conversion1 : DataTypeConversion  OutDataTypeStr=uint8
  Data Type Conversion2 : DataTypeConversion  OutDataTypeStr=uint8
  Detect Decrease : simulink/Logic and Bit Operations/Detect Decrease  vinit=0.0  OutDataTypeStr=boolean
  Detect Decrease1 : simulink/Logic and Bit Operations/Detect Decrease  vinit=0.0  OutDataTypeStr=boolean
  Detect Increase : simulink/Logic and Bit Operations/Detect Increase  vinit=0.0  OutDataTypeStr=boolean
  Detect Increase1 : simulink/Logic and Bit Operations/Detect Increase  vinit=0.0  OutDataTypeStr=boolean
  Equal{,1..2,4..6,8..22,24..28,30..31,33..34} (30 alike) : RelationalOperator  Operator===  OutDataTypeStr=boolean  RndMeth=Simplest
  Equal23 : RelationalOperator  Operator=~=  OutDataTypeStr=boolean  RndMeth=Simplest
  Equal29 : RelationalOperator  OutDataTypeStr=boolean  RndMeth=Simplest
  Equal3 : RelationalOperator  Operator=~=  OutDataTypeStr=boolean  RndMeth=Simplest
  Equal7 : RelationalOperator  OutDataTypeStr=boolean  RndMeth=Simplest
  Logical Operator{,4,6,8,10..11,21,25,27,77} (10 alike) : Logic  Operator=OR  AllPortsSameDT=off  OutDataTypeStr=boolean
  Logical Operator{1..2,9,13,15..18,24,55} (10 alike) : Logic  AllPortsSameDT=off  OutDataTypeStr=boolean
  Logical Operator{12,14,28..31} (6 alike) : Logic  Operator=NOT  AllPortsSameDT=off  OutDataTypeStr=boolean
  Logical Operator{3,5,19,23} (4 alike) : Logic  Inputs=8  AllPortsSameDT=off  OutDataTypeStr=boolean
  Logical Operator20 : Logic  Operator=OR  Inputs=3  AllPortsSameDT=off  OutDataTypeStr=boolean
  Logical Operator{7,22,26,40} (4 alike) : Logic  Operator=OR  Inputs=4  AllPortsSameDT=off  OutDataTypeStr=boolean
  Logical Operator37 : Logic  Operator=OR  Inputs=3  AllPortsSameDT=off  OutDataTypeStr=boolean
  Relay1 : Relay  OnSwitchValue=ONE_INT  OffSwitchValue=ZERO_INT
  Relay2 : Relay  OnSwitchValue=ONE_INT  OffSwitchValue=ZERO_INT
  SR_Latch{1..5,12} (6 alike) : hcu_lib/Basic_Blocks/SR_Latch
  Switch1 : Switch  Criteria=u2 ~= 0
  Switch6 : Switch  Criteria=u2 ~= 0
  Test Detection Criteria1 : hcu_lib/Basic_Blocks/Test Detection Criteria
  Test Detection Criteria2 : hcu_lib/Basic_Blocks/Test Detection Criteria
  Timer1 : hcu_lib/Basic_Blocks/Timer
  Timer2 : hcu_lib/Basic_Blocks/Timer
  Unit Delay{,1..2,4} (4 alike) : UnitDelay  SampleTime=-1  HasFrameUpgradeWarning=on
  VDDM_EPBLockTODTC_raw32 : Outport
  VDDM_EPBUnlockTODTC_raw32 : Outport  Port=2
  wires:
  [VDDM_EPBLockTODTC_cnt] -> Relay1/1
  [VDDM_EPBLockTOCFS_flg] -> Logical Operator77/2
  [VDDM_EPBLockTORst_flg] -> SR_Latch12/2
  Switch6/1 -> Test Detection Criteria1/1
  Constant21/1 -> Equal7/2
  [VDDM_EPBLockTODFSRls_flg] -> Logical Operator77/1
  DTC_Couter1/1 -> SR_Latch1/1
  Logical Operator15/1 -> DTC_Couter1/1
  [VDDM_EPBLockTOPass_flg] -> DTC_Info/2
  Logical Operator3/1 -> [VDDM_EPBLockTORst_flg], Switch6/3
  Constant22/1 -> Test Detection Criteria1/4
  [VDDM_EPBLockTOCFSRls_flg] -> SR_Latch1/2
  Constant2/1 -> Switch6/1
  Equal7/1 -> SR_Latch12/1
  Logical Operator2/1 -> [VDDM_EPBLockTOCFS_flg]
  Constant20/1 -> Test Detection Criteria1/3
  Data Type Conversion2/1 -> [VDDM_EPBLockTODTC_cnt]  "VDDM_EPBLockTODTC_cnt"
  Timer2/1 -> Equal7/1
  DTC_Couter1/2 -> Data Type Conversion2/1
  [VDDM_EPBLockTOCFS_flg] -> DTC_Info/3
  [VDDM_EPBLockTODet_flg] -> DTC_Info/1
  [task_time_s] -> Test Detection Criteria1/2
  Relay1/1 -> SR_Latch2/1
  Logical Operator77/1 -> SR_Latch2/2
  DTC_Info/1 -> VDDM_EPBLockTODTC_raw32/1  "VDDM_EPBLockTODTC_raw32"
  Test Detection Criteria1/1 -> [VDDM_EPBLockTODet_flg]  "VDDM_EPBLockTODet_flg"
  Constant16/1 -> Logical Operator55/1
  Constant6/1 -> Logical Operator15/2
  Logical Operator55/1 -> [VDDM_EPBLockTODFS_flg]
  [DTC_clear_request] -> Switch6/2
  Constant70/1 -> Timer2/4
  Logical Operator11/1 -> Logical Operator16/1
  SR_Latch1/1 -> Logical Operator2/1
  [VDDM_EPBLockTOPass_flg] -> Logical Operator11/1
  Constant1/1 -> Logical Operator2/2
  [VDDM_EPBLockTOCFSRls_flg] -> Logical Operator11/2
  Constant7/1 -> Logical Operator16/2
  SR_Latch12/1 -> [VDDM_EPBLockTOPass_flg]
  [DTC_clear_request] -> DTC_Info/4
  Logical Operator14/1 -> Timer2/2
  Logical Operator5/1 -> Logical Operator14/1, Timer2/1
  [VDDM_EPBLockTODet_flg] -> Logical Operator15/1
  [task_time_s] -> Timer2/3
  Logical Operator16/1 -> DTC_Couter1/2
  Constant15/1 -> DTC_Couter1/3
  SR_Latch2/1 -> Logical Operator55/2
  [VPMM_SysPwrSta_enum] -> Equal1/1
  Constant9/1 -> Equal3/2
  Detect Increase/1 -> Logical Operator3/7
  [NO_CS_LossErrOfEPB1] -> Logical Operator3/4
  [VINP_EPBSta_enum] -> Equal3/1
  [VDDM_EPBUnlockTOCFS_flg] -> Unit Delay/1
  Equal3/1 -> Logical Operator3/8
  [VDDM_ParkRequest_flg] -> Detect Increase/1
  Constant8/1 -> Equal1/2
  Logical Operator/1 -> Logical Operator3/5
  [NO_RC_LossErrOfEPB1] -> Logical Operator3/3
  [NO_CAN1_BUS_OFF] -> Logical Operator3/1
  Equal1/1 -> Logical Operator/2
  Equal/1 -> Logical Operator/1
  Constant/1 -> Equal/2
  [VPMM_SysPwrSta_enum] -> Equal/1
  [NO_CAN_LossOfEPB1] -> Logical Operator3/2
  Detect Increase1/1 -> Logical Operator5/7
  Equal4/1 -> Logical Operator4/2
  [NO_CAN1_BUS_OFF] -> Logical Operator5/1
  Equal2/1 -> Logical Operator4/1
  [VPMM_SysPwrSta_enum] -> Equal2/1
  Constant3/1 -> Equal2/2
  [VDDM_EPBUnlockTOCFS_flg] -> Unit Delay2/1
  [NO_CAN_LossOfEPB1] -> Logical Operator5/2
  Logical Operator4/1 -> Logical Operator5/5
  [VINP_EPBSta_enum] -> Equal5/1
  Constant11/1 -> Equal5/2
  Constant10/1 -> Equal4/2
  [NO_CS_LossErrOfEPB1] -> Logical Operator5/4
  [VPMM_SysPwrSta_enum] -> Equal4/1
  Equal5/1 -> Logical Operator5/8
  [VDDM_ParkRequest_flg] -> Detect Increase1/1
  [NO_RC_LossErrOfEPB1] -> Logical Operator5/3
  Equal10/1 -> Logical Operator1/2
  Constant45/1 -> Equal33/2
  Logical Operator1/1 -> Logical Operator37/2
  Equal33/1 -> Logical Operator40/1
  [VINP_ShifterHandleCmd_enum] -> Equal6/1
  Constant46/1 -> Equal34/2
  Constant12/1 -> Equal9/2
  [VPMM_SysPwrSta_enum] -> Equal10/1
  [DTC_clear_request] -> Logical Operator37/3
  Unit Delay4/1 -> Equal9/1
  Constant13/1 -> Equal10/2
  Equal8/1 -> Logical Operator40/4
  [VPMM_SysPwrSta_enum] -> Unit Delay4/1
  Constant4/1 -> Equal6/2
  Equal9/1 -> Logical Operator1/1
  Logical Operator40/1 -> Logical Operator37/1
  Constant5/1 -> Equal8/2
  [VINP_ShifterHandleCmd_enum] -> Equal33/1
  Equal6/1 -> Logical Operator40/3
  [VINP_ShifterHandleCmd_enum] -> Equal34/1
  Equal34/1 -> Logical Operator40/2
  Logical Operator37/1 -> [VDDM_EPBLockTOCFSRls_flg]
  [VINP_ShifterHandleCmd_enum] -> Equal8/1
  Constant18/1 -> Equal13/2
  Equal13/1 -> Logical Operator7/3
  [VINP_ShifterHandleCmd_enum] -> Equal12/1
  Constant19/1 -> Equal14/2
  Equal14/1 -> Logical Operator7/4
  [VINP_ShifterHandleCmd_enum] -> Equal11/1
  [VINP_ShifterHandleCmd_enum] -> Equal13/1
  Equal11/1 -> Logical Operator7/1
  Constant14/1 -> Equal11/2
  Logical Operator6/1 -> [VDDM_EPBLockTODFSRls_flg]
  [VINP_ShifterHandleCmd_enum] -> Equal14/1
  Equal12/1 -> Logical Operator7/2
  Constant17/1 -> Equal12/2
  [VDDM_EPBLockTOPass_flg] -> Logical Operator6/2
  Logical Operator7/1 -> Logical Operator6/1
  Detect Decrease1/1 -> Logical Operator23/7
  [VDDM_ParkRequest_flg] -> Detect Decrease1/1
  Logical Operator28/1 -> Logical Operator19/6
  [VDDM_EPBUnlockTODFSRls_flg] -> Logical Operator27/1
  Detect Decrease/1 -> Logical Operator19/7
  [VDDM_EPBUnlockTODTC_cnt] -> Relay2/1
  Equal29/1 -> SR_Latch4/1
  Logical Operator19/1 -> [VDDM_EPBUnlockTORst_flg], Switch1/3
  Constant37/1 -> Equal29/2
  [VDDM_EPBUnlockTODet_flg] -> DTC_Info1/1
  [NO_RC_LossErrOfEPB1] -> Logical Operator23/3
  DTC_Info1/1 -> VDDM_EPBUnlockTODTC_raw32/1  "VDDM_EPBUnlockTODTC_raw32"
  Constant48/1 -> Timer1/4
  [NO_CAN1_BUS_OFF] -> Logical Operator23/1
  Logical Operator10/1 -> Logical Operator17/1
  Logical Operator24/1 -> [VDDM_EPBUnlockTODFS_flg]
  SR_Latch4/1 -> [VDDM_EPBUnlockTOPass_flg]
  Switch1/1 -> Test Detection Criteria2/1
  [VDDM_EPBUnlockTOCFSRls_flg] -> SR_Latch3/2
  [DTC_clear_request] -> Logical Operator20/3
  Constant36/1 -> Test Detection Criteria2/3
  Constant50/1 -> Equal23/2
  Timer1/1 -> Equal29/1
  [VDDM_EPBUnlockTOPass_flg] -> Logical Operator10/1
  [VDDM_EPBUnlockTOCFSRls_flg] -> Logical Operator10/2
  DTC_Couter2/2 -> Data Type Conversion1/1
  Relay2/1 -> SR_Latch5/1
  [VDDM_EPBUnlockTOCFS_flg] -> DTC_Info1/3
  Logical Operator18/1 -> [VDDM_EPBUnlockTOCFS_flg]
  [NO_RC_LossErrOfEPB1] -> Logical Operator19/3
  Equal26/1 -> Logical Operator21/2
  Logical Operator12/1 -> Timer1/2
  Equal23/1 -> Logical Operator19/8
  Logical Operator17/1 -> DTC_Couter2/2
  Logical Operator8/1 -> Logical Operator19/5
  DTC_Couter2/1 -> SR_Latch3/1
  Constant44/1 -> Logical Operator13/2
  Logical Operator13/1 -> DTC_Couter2/1
  Constant31/1 -> Logical Operator24/1
  Constant23/1 -> Equal15/2
  Data Type Conversion1/1 -> [VDDM_EPBUnlockTODTC_cnt]  "VDDM_EPBUnlockTODTC_cnt"
  SR_Latch5/1 -> Logical Operator24/2
  [VPMM_SysPwrSta_enum] -> Equal15/1
  [DTC_clear_request] -> DTC_Info1/4
  [VPMM_SysPwrSta_enum] -> Equal22/1
  Constant39/1 -> Equal22/2
  [VDDM_EPBLockTOCFS_flg] -> Logical Operator28/1
  Constant41/1 -> Equal24/2
  Unit Delay1/1 -> Equal31/1
  [NO_CAN_LossOfEPB1] -> Logical Operator23/2
  Equal15/1 -> Logical Operator8/1
  Equal22/1 -> Logical Operator21/1
  [NO_CAN_LossOfEPB1] -> Logical Operator19/2
  Constant38/1 -> Test Detection Criteria2/4
  [VINP_ShifterHandleCmd_enum] -> Equal25/1
  Equal24/1 -> Logical Operator22/1
  [VDDM_EPBUnlockTOCFS_flg] -> Logical Operator27/2
  [DTC_clear_request] -> Switch1/2
  Equal30/1 -> Logical Operator22/4
  Equal27/1 -> Logical Operator23/8
  Constant30/1 -> DTC_Couter2/3
  Logical Operator23/1 -> Logical Operator12/1, Timer1/1
  Equal17/1 -> Logical Operator9/2
  Constant27/1 -> Equal31/2
  Equal25/1 -> Logical Operator22/2
  SR_Latch3/1 -> Logical Operator18/1
  Logical Operator22/1 -> Logical Operator20/1
  [VPMM_SysPwrSta_enum] -> Equal26/1
  [VINP_EPBSta_enum] -> Equal27/1
  Equal31/1 -> Logical Operator9/1
  [VINP_ShifterHandleCmd_enum] -> Equal24/1
  Constant33/1 -> Equal20/2
  Equal28/1 -> Logical Operator22/3
  Constant40/1 -> Equal28/2
  Equal21/1 -> Logical Operator26/4
  Constant26/1 -> Equal27/2
  [VDDM_EPBUnlockTODet_flg] -> Logical Operator13/1
  Logical Operator20/1 -> [VDDM_EPBUnlockTOCFSRls_flg]
  [VINP_ShifterHandleCmd_enum] -> Equal30/1
  [NO_CS_LossErrOfEPB1] -> Logical Operator23/4
  Constant42/1 -> Equal25/2
  Equal20/1 -> Logical Operator26/3
  Logical Operator9/1 -> Logical Operator20/2
  Logical Operator27/1 -> SR_Latch5/2
  Equal16/1 -> Logical Operator8/2
  Constant28/1 -> Equal17/2
  [VINP_ShifterHandleCmd_enum] -> Equal28/1
  [VINP_ShifterHandleCmd_enum] -> Equal20/1
  Constant32/1 -> Equal19/2
  [VPMM_SysPwrSta_enum] -> Equal17/1
  [task_time_s] -> Timer1/3
  Test Detection Criteria2/1 -> [VDDM_EPBUnlockTODet_flg]  "VDDM_EPBUnlockTODet_flg"
  [VDDM_EPBLockTOCFS_flg] -> Logical Operator29/1
  [NO_CAN1_BUS_OFF] -> Logical Operator19/1
  Constant49/1 -> Equal16/2
  [VINP_EPBSta_enum] -> Equal23/1
  [VDDM_EPBUnlockTOPass_flg] -> Logical Operator25/2
  Constant34/1 -> Equal21/2
  Equal19/1 -> Logical Operator26/2
  Constant25/1 -> Equal26/2
  [VPMM_SysPwrSta_enum] -> Unit Delay1/1
  [NO_CS_LossErrOfEPB1] -> Logical Operator19/4
  Logical Operator25/1 -> [VDDM_EPBUnlockTODFSRls_flg]
  Constant43/1 -> Equal30/2
  [VINP_ShifterHandleCmd_enum] -> Equal18/1
  Constant47/1 -> Logical Operator17/2
  Constant35/1 -> Switch1/1
  Logical Operator26/1 -> Logical Operator25/1
  Equal18/1 -> Logical Operator26/1
  [VINP_ShifterHandleCmd_enum] -> Equal19/1
  [VPMM_SysPwrSta_enum] -> Equal16/1
  [task_time_s] -> Test Detection Criteria2/2
  Constant24/1 -> Logical Operator18/2
  [VINP_ShifterHandleCmd_enum] -> Equal21/1
  [VDDM_EPBUnlockTORst_flg] -> SR_Latch4/2
  Constant29/1 -> Equal18/2
  Logical Operator29/1 -> Logical Operator23/6
  [VDDM_ParkRequest_flg] -> Detect Decrease/1
  [VDDM_EPBUnlockTOPass_flg] -> DTC_Info1/2
  Logical Operator21/1 -> Logical Operator23/5
  Logical Operator30/1 -> Logical Operator3/6
  Logical Operator31/1 -> Logical Operator5/6
  Unit Delay/1 -> Logical Operator30/1
  Unit Delay2/1 -> Logical Operator31/1
